simulink model "rotpentemplate"  (R2025b)
settings: Solver=ode45  StartTime=0.0  StopTime=60  RelTol=1e-3  EnableMultiTasking=on
undefined symbols (not defined in the file): p_identified, u_down, x_down
settings Model: Creator=rbabuska  LastModifiedBy=thoma
settings SolverCC: AlgebraicLoopSolver=TrustRegion
settings DataIOCC: LimitDataPoints=on  SaveFormat=Array  ReturnWorkspaceOutputs=off  SignalLoggingName=sigsOut
settings OptimizationCC: BooleanDataType=off  ExpressionDepthLimit=2147483647.0  InitFltsAndDblsToZero=on  LifeSpan=inf
settings DebuggingCC: SaveWithParameterizedLinksMsg=none  SignalResolutionControl=TryResolveAllWithWarning  MultiTaskDSMMsg=warning  MultiTaskCondExecSysMsg=none  UnconnectedInputMsg=warning  UnconnectedOutputMsg=warning  UnconnectedLineMsg=warning  AllowSymbolicDim=off  StateNameClashWarn=warning  SFUnexpectedBacktrackingDiag=warning  SFNoUnconditionalDefaultTransitionDiag=warning  SFExecutionAtInitializationDiag=none  ArithmeticOperatorsInVariantConditions=warning
settings HardwareCC: ProdBitPerPointer=32.0  ProdBitPerSizeT=32.0  ProdBitPerPtrDiffT=32.0  ProdLargestAtomicFloat=None  ProdIntDivRoundTo=Undefined  ProdEndianess=Unspecified  ProdWordSize=32.0  ProdHWDeviceType=32-bit Generic  TargetUnknown=on
settings ModelReferenceCC: EnableRefExpFcnMdlSchedulingChecks=on  PropagateSignalLabelsOutOfModel=off
settings SFSimCC: SimUseLocalCustomCode=off  CustomCodeUndefinedFunction=UseInterfaceOnly
settings RTWCC: RTWUseLocalCustomCode=off  GPUComputeCapability=3.5
settings CodeAppCC: StateflowObjectComments=on
settings GRTTargetCC: TargetFcnLib=ansi_tfl_tmw.mat  TargetLangStandard=C89/C90 (ANSI)  CombineOutputUpdateFcns=off  GRTInterface=on
settings ConfigComp: CovMetricSettings=dw  CovSaveCumulativeToWorkspaceVar=on  CovSaveSingleToWorkspaceVar=on  CovExternalEMLEnable=off

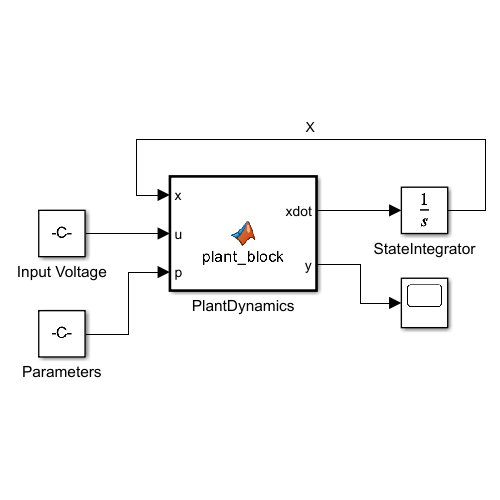
[thumbnail: Simulink's stored preview of the top-level diagram]
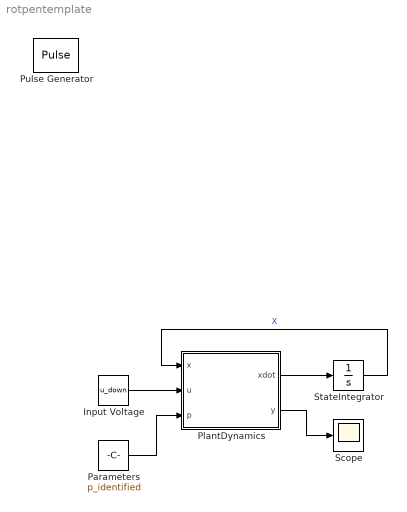
== system rotpentemplate ==
  Input Voltage : Constant  Value=u_down
  Parameters : Constant  Value=p_identified
  PlantDynamics : MATLAB Function  TreatAsAtomicUnit=on
  Scope : Scope
      settings: ActiveDisplayYMinimum=-6.3017858690225506  ActiveDisplayYMaximum=12.41009552166553  DataLoggingVariableName=ScopeData3
  StateIntegrator : Integrator  InitialCondition=x_down
  Pulse Generator : DiscretePulseGenerator  IOType=siggen  PulseType=Time based  PulseWidth=50
  wires:
  Parameters/1 -> PlantDynamics/3(p)
  Input Voltage/1 -> PlantDynamics/2(u)
  PlantDynamics/1(xdot) -> StateIntegrator/1
  StateIntegrator/1 -> PlantDynamics/1(x)  "X"
  PlantDynamics/2(y) -> Scope/1

== matlab function rotpentemplate/PlantDynamics ==
  data: x input; xdot output; u input; y output; p input
function [xdot, y] = plant_block(x, u, p)
%#codegen

[xdot, y] = pendulum_nonlinear_rhs(x, u, p);

end
